simulink library "scdexblks"  (Simulink 7.6)
settings: Solver=ode45  SolverMode=SingleTasking  StartTime=0.0  StopTime=10.0  RelTol=1e-3
settings Model: Creator=The MathWorks Inc.

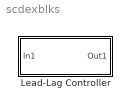
== system scdexblks ==
  Lead-Lag Controller : Subsystem  SCDConfigFcn=scdleadexample  mask(Lead-Lag Controller){Gain=100, Zero=15, Pole=50}
      mask prompts: Zero "Zero Frequency (rad/s)"; Pole "Pole Frequency (rad/s)"
      mask help: This block implements a lead-lag controller which consists of 1 zero, 1 pole, and a gain.
      mask Display: fprintf('Lead-Lag Ctrl');

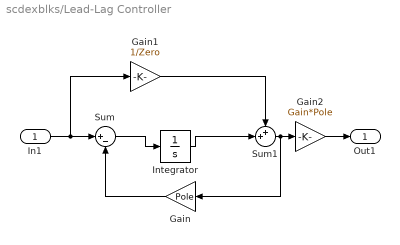
== system scdexblks/Lead-Lag Controller ==
  In1 : Inport
  Gain : Gain  Gain=Pole
  Gain1 : Gain  Gain=1/Zero
  Gain2 : Gain  Gain=Gain*Pole
  Integrator : Integrator
  Sum : Sum  Inputs=|+-
  Sum1 : Sum  Inputs=++|
  Out1 : Outport
  wires:
  Sum1/1 -> Gain/1, Gain2/1
  Integrator/1 -> Sum1/2
  Gain1/1 -> Sum1/1
  Sum/1 -> Integrator/1
  In1/1 -> Sum/1, Gain1/1
  Gain/1 -> Sum/2
  Gain2/1 -> Out1/1
